simulink model "ValidateThrustersRED"  (R2020a)
settings: Solver=FixedStepAuto  StartTime=0.0  StopTime=tsim  RelTol=1e-3  EnableMultiTasking=on
undefined symbols (not defined in the file): Thruster1_OnTime, Thruster2_OnTime, Thruster3_OnTime, Thruster4_OnTime, Thruster5_OnTime, Thruster6_OnTime, Thruster7_OnTime, Thruster8_OnTime, ThrusterOff_Time
libraries: raspberrypiBasiclib x9
settings Model: SimulationMode=external  ExtModeTrigDuration=2  Creator=AlexC  LastModifiedBy=SPOT
settings SolverCC: PositivePriorityOrder=on
settings DataIOCC: ReturnWorkspaceOutputs=off
settings OptimizationCC: MaxStackSize=64
settings DebuggingCC: ParameterTunabilityLossMsg=error  ArithmeticOperatorsInVariantConditions=warning
settings HardwareCC: ProdBitPerPointer=32  ProdBitPerSizeT=32  ProdBitPerPtrDiffT=32  ProdLargestAtomicInteger=Long  ProdLargestAtomicFloat=Double  ProdWordSize=32  ProdHWDeviceType=ARM Compatible->ARM Cortex  UseEmbeddedCoderFeatures=off
settings SFSimCC: SimUseLocalCustomCode=off  CustomCodeUndefinedFunction=UseInterfaceOnly
settings RTWCC: SystemTargetFile=ert.tlc  HardwareBoard=Raspberry Pi  TemplateMakefile=ert_default_tmf  GenerateReport=on  RTWUseLocalCustomCode=off  Toolchain=GNU GCC Raspberry Pi  BuildConfiguration=Faster Runs  LaunchReport=on
settings CodeAppCC: ForceParamTrailComments=on  OperatorAnnotations=on  StateflowObjectComments=on  MATLABSourceComments=on
settings ERTTargetCC: ERTCustomFileBanners=off  MatFileLogging=on  SupportContinuousTime=on  SupportNonInlinedSFcns=on  RemoveResetFunc=off  SupportVariableSizeSignals=on  ModelStepFunctionPrototypeControlCompliant=off

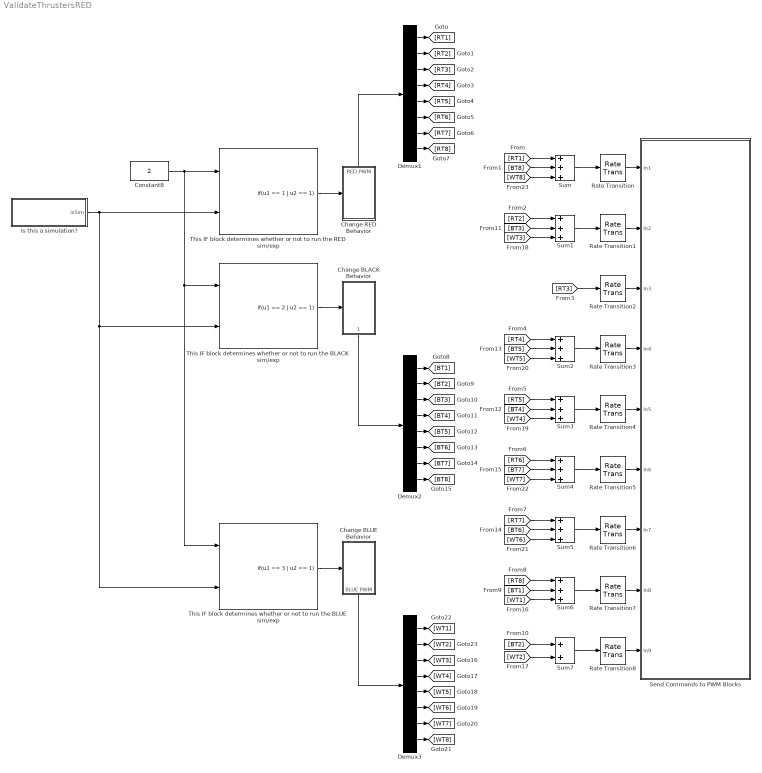
== system ValidateThrustersRED ==
  Change BLACK Behavior : Subsystem  TreatAsAtomicUnit=on
  Change BLUE Behavior : Subsystem  TreatAsAtomicUnit=on
  Change RED Behavior : Subsystem  TreatAsAtomicUnit=on
  Constant8 : Constant  Value=2
  Demux1 : Demux  Outputs=8
  Demux2 : Demux  Outputs=8
  Demux3 : Demux  Outputs=8
  Is this a simulation? : Subsystem
  Rate Transition{,1..8} (9 alike) : RateTransition  OutPortSampleTime=0.1
  Send Commands to PWM Blocks : Subsystem  TreatAsAtomicUnit=on  SystemSampleTime=0.1
  Sum{,1..6} (7 alike) : Sum  Inputs=+++
  Sum7 : Sum
  This IF block determines whether or not to run the BLACK sim/exp : If  NumInputs=2  IfExpression=u1 == 2 | u2 == 1  ShowElse=off
  This IF block determines whether or not to run the BLUE sim/exp : If  NumInputs=2  IfExpression=u1 == 3 | u2 == 1  ShowElse=off
  "This IF block determines whether or not to run the RED sim/exp " : If  NumInputs=2  IfExpression=u1 == 1 | u2 == 1  ShowElse=off
  wires:
  Demux3/8 -> [WT8]
  Rate Transition2/1 -> Send Commands to PWM Blocks/3(In3)
  Sum6/1 -> Rate Transition7/1
  This IF block determines whether or not to run the BLUE sim/exp/1 -> Change BLUE Behavior/Action
  Demux2/2 -> [BT2]
  This IF block determines whether or not to run the BLACK sim/exp/1 -> Change BLACK Behavior/Action
  Constant8/1 -> This IF block determines whether or not to run the BLUE sim/exp/1, This IF block determines whether or not to run the BLACK sim/exp/1, "This IF block determines whether or not to run the RED sim/exp "/1
  Demux2/4 -> [BT4]
  Rate Transition5/1 -> Send Commands to PWM Blocks/6(In6)
  Demux3/4 -> [WT4]
  Rate Transition8/1 -> Send Commands to PWM Blocks/9(In9)
  Demux3/7 -> [WT7]
  [RT4] -> Sum2/1
  Rate Transition7/1 -> Send Commands to PWM Blocks/8(In8)
  Sum4/1 -> Rate Transition5/1
  Demux1/7 -> [RT7]
  Demux3/6 -> [WT6]
  Demux1/8 -> [RT8]
  Demux1/3 -> [RT3]
  Sum3/1 -> Rate Transition4/1
  Sum5/1 -> Rate Transition6/1
  Sum2/1 -> Rate Transition3/1
  Change RED Behavior/1(RED PWM) -> Demux1/1
  [BT5] -> Sum2/2
  [BT7] -> Sum4/2
  [BT3] -> Sum1/2
  [RT2] -> Sum1/1
  [BT6] -> Sum5/2
  [BT8] -> Sum/2
  [RT7] -> Sum5/1
  Rate Transition3/1 -> Send Commands to PWM Blocks/4(In4)
  Change BLACK Behavior/1(BLACK PWM) -> Demux2/1
  Demux2/3 -> [BT3]
  Demux2/6 -> [BT6]
  Demux1/6 -> [RT6]
  [BT1] -> Sum6/2
  Demux2/7 -> [BT7]
  Demux1/4 -> [RT4]
  Is this a simulation?/1(isSim) -> This IF block determines whether or not to run the BLACK sim/exp/2, This IF block determines whether or not to run the BLUE sim/exp/2, "This IF block determines whether or not to run the RED sim/exp "/2
  Rate Transition4/1 -> Send Commands to PWM Blocks/5(In5)
  Demux2/5 -> [BT5]
  [WT3] -> Sum1/3
  Demux3/5 -> [WT5]
  Demux1/2 -> [RT2]
  [RT1] -> Sum/1
  [WT1] -> Sum6/3
  Demux3/3 -> [WT3]
  Sum/1 -> Rate Transition/1
  Sum7/1 -> Rate Transition8/1
  Demux2/8 -> [BT8]
  [RT8] -> Sum6/1
  [BT4] -> Sum3/2
  Change BLUE Behavior/1(BLUE PWM) -> Demux3/1
  Rate Transition6/1 -> Send Commands to PWM Blocks/7(In7)
  Demux1/5 -> [RT5]
  [RT5] -> Sum3/1
  Demux3/1 -> [WT1]
  Demux2/1 -> [BT1]
  [WT6] -> Sum5/3
  [WT2] -> Sum7/2
  "This IF block determines whether or not to run the RED sim/exp "/1 -> Change RED Behavior/Action
  [WT7] -> Sum4/3
  [RT6] -> Sum4/1
  [WT5] -> Sum2/3
  Sum1/1 -> Rate Transition1/1
  Demux3/2 -> [WT2]
  [BT2] -> Sum7/1
  [WT4] -> Sum3/3
  Demux1/1 -> [RT1]
  Rate Transition/1 -> Send Commands to PWM Blocks/1(In1)
  [WT8] -> Sum/3
  [RT3] -> Rate Transition2/1
  Rate Transition1/1 -> Send Commands to PWM Blocks/2(In2)

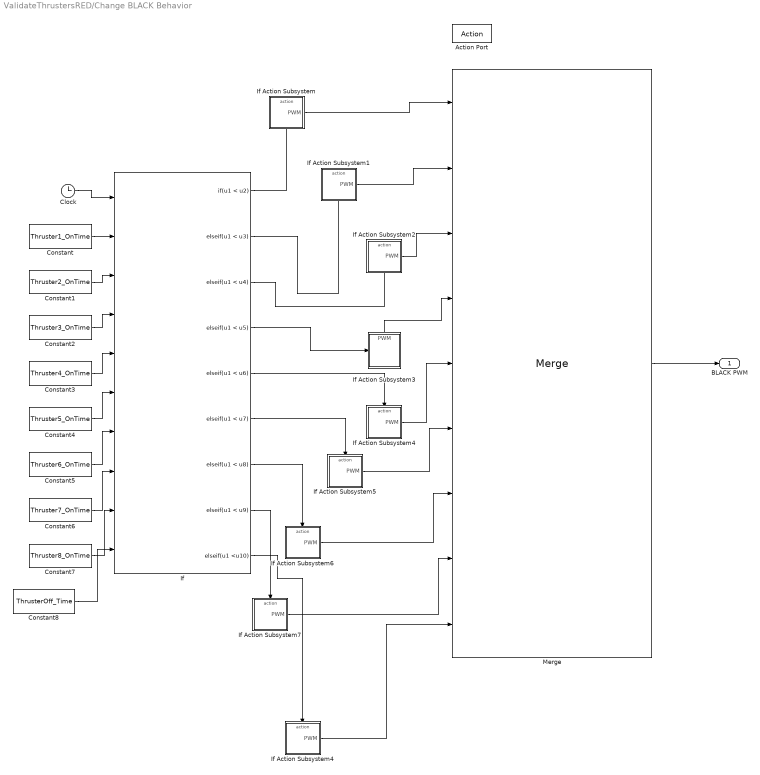
== system ValidateThrustersRED/Change BLACK Behavior ==
  Action Port : ActionPort  ActionPortLabel=if(u1 == 2 | u2 == 1)
  Clock : Clock
  Constant : Constant  Value=Thruster1_OnTime
  Constant1 : Constant  Value=Thruster2_OnTime
  Constant2 : Constant  Value=Thruster3_OnTime
  Constant3 : Constant  Value=Thruster4_OnTime
  Constant4 : Constant  Value=Thruster5_OnTime
  Constant5 : Constant  Value=Thruster6_OnTime
  Constant6 : Constant  Value=Thruster7_OnTime
  Constant7 : Constant  Value=Thruster8_OnTime
  Constant8 : Constant  Value=ThrusterOff_Time
  If : If  NumInputs=10  IfExpression=u1 < u2  ElseIfExpressions=u1 < u3, u1 < u4, u1 < u5, u1 < u6, u1 < u7, u1 < u8, u1 < u9, u1 <u10  ShowElse=off
  If Action Subsystem : Subsystem  TreatAsAtomicUnit=on
  If Action Subsystem1 : Subsystem  TreatAsAtomicUnit=on
  If Action Subsystem2 : Subsystem  TreatAsAtomicUnit=on
  If Action Subsystem3 : Subsystem  TreatAsAtomicUnit=on
  If Action Subsystem4 : Subsystem  TreatAsAtomicUnit=on
  If Action Subsystem5 : Subsystem  TreatAsAtomicUnit=on
  If Action Subsystem6 : Subsystem  TreatAsAtomicUnit=on
  If Action Subsystem7 : Subsystem  TreatAsAtomicUnit=on
  If Action Subsystem4 : Subsystem  TreatAsAtomicUnit=on
  Merge : Merge  Inputs=9
  BLACK PWM : Outport  VectorParamsAs1DForOutWhenUnconnected=off
  wires:
  Merge/1 -> BLACK PWM/1
  If/7 -> If Action Subsystem6/Action
  Constant6/1 -> If/8
  If/3 -> If Action Subsystem2/Action
  Constant4/1 -> If/6
  Constant3/1 -> If/5
  If Action Subsystem1/1(PWM) -> Merge/2
  If Action Subsystem2/1(PWM) -> Merge/3
  Constant/1 -> If/2
  Constant5/1 -> If/7
  Constant2/1 -> If/4
  If/5 -> If Action Subsystem4/Action
  If/6 -> If Action Subsystem5/Action
  If/8 -> If Action Subsystem7/Action
  Constant7/1 -> If/9
  If/2 -> If Action Subsystem1/Action
  If Action Subsystem4/1(PWM) -> Merge/5
  If Action Subsystem5/1(PWM) -> Merge/6
  If/4 -> If Action Subsystem3/Action
  If Action Subsystem/1(PWM) -> Merge/1
  If/1 -> If Action Subsystem/Action
  Clock/1 -> If/1
  Constant1/1 -> If/3
  If Action Subsystem6/1(PWM) -> Merge/7
  If Action Subsystem7/1(PWM) -> Merge/8
  If Action Subsystem3/1(PWM) -> Merge/4
  Constant8/1 -> If/10
  If Action Subsystem4/1(PWM) -> Merge/9
  If/9 -> If Action Subsystem4/Action

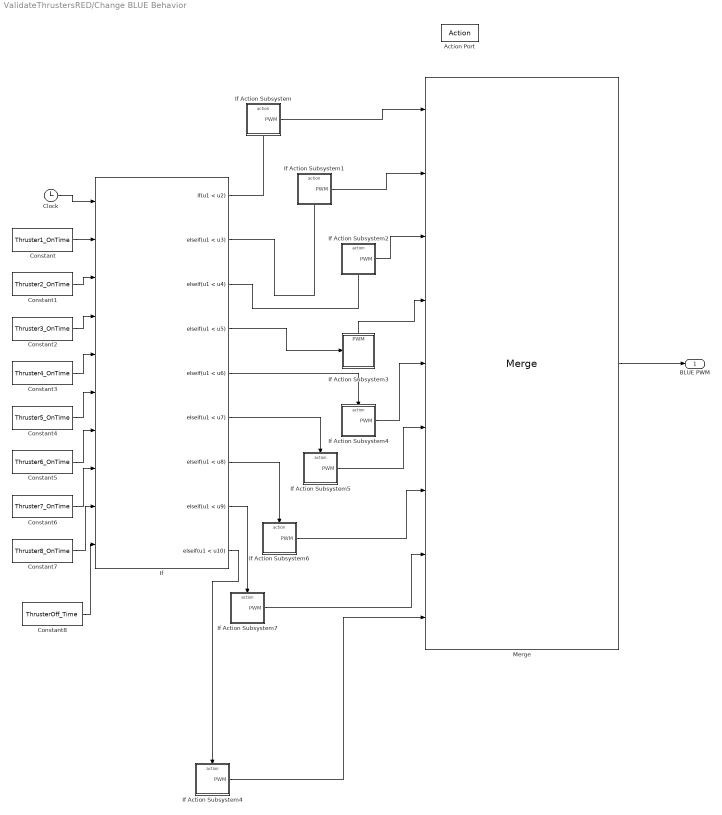
== system ValidateThrustersRED/Change BLUE Behavior ==
  Action Port : ActionPort  ActionPortLabel=if(u1 == 3 | u2 == 1)
  Clock : Clock
  Constant : Constant  Value=Thruster1_OnTime
  Constant1 : Constant  Value=Thruster2_OnTime
  Constant2 : Constant  Value=Thruster3_OnTime
  Constant3 : Constant  Value=Thruster4_OnTime
  Constant4 : Constant  Value=Thruster5_OnTime
  Constant5 : Constant  Value=Thruster6_OnTime
  Constant6 : Constant  Value=Thruster7_OnTime
  Constant7 : Constant  Value=Thruster8_OnTime
  Constant8 : Constant  Value=ThrusterOff_Time
  If : If  NumInputs=10  IfExpression=u1 < u2  ElseIfExpressions=u1 < u3, u1 < u4, u1 < u5, u1 < u6, u1 < u7, u1 < u8, u1 < u9, u1 < u10  ShowElse=off
  If Action Subsystem : Subsystem  TreatAsAtomicUnit=on
  If Action Subsystem1 : Subsystem  TreatAsAtomicUnit=on
  If Action Subsystem2 : Subsystem  TreatAsAtomicUnit=on
  If Action Subsystem3 : Subsystem  TreatAsAtomicUnit=on
  If Action Subsystem4 : Subsystem  TreatAsAtomicUnit=on
  If Action Subsystem5 : Subsystem  TreatAsAtomicUnit=on
  If Action Subsystem6 : Subsystem  TreatAsAtomicUnit=on
  If Action Subsystem7 : Subsystem  TreatAsAtomicUnit=on
  If Action Subsystem4 : Subsystem  TreatAsAtomicUnit=on
  Merge : Merge  Inputs=9
  BLUE PWM : Outport  VectorParamsAs1DForOutWhenUnconnected=off
  wires:
  Merge/1 -> BLUE PWM/1
  If/7 -> If Action Subsystem6/Action
  Constant6/1 -> If/8
  If/3 -> If Action Subsystem2/Action
  Constant4/1 -> If/6
  Constant3/1 -> If/5
  If Action Subsystem1/1(PWM) -> Merge/2
  If Action Subsystem2/1(PWM) -> Merge/3
  Constant/1 -> If/2
  Constant5/1 -> If/7
  Constant2/1 -> If/4
  If/5 -> If Action Subsystem4/Action
  If/6 -> If Action Subsystem5/Action
  If/8 -> If Action Subsystem7/Action
  Constant7/1 -> If/9
  If/2 -> If Action Subsystem1/Action
  If Action Subsystem4/1(PWM) -> Merge/5
  If Action Subsystem5/1(PWM) -> Merge/6
  If/4 -> If Action Subsystem3/Action
  If Action Subsystem/1(PWM) -> Merge/1
  If/1 -> If Action Subsystem/Action
  Clock/1 -> If/1
  Constant1/1 -> If/3
  If Action Subsystem6/1(PWM) -> Merge/7
  If Action Subsystem7/1(PWM) -> Merge/8
  If Action Subsystem3/1(PWM) -> Merge/4
  If Action Subsystem4/1(PWM) -> Merge/9
  If/9 -> If Action Subsystem4/Action
  Constant8/1 -> If/10

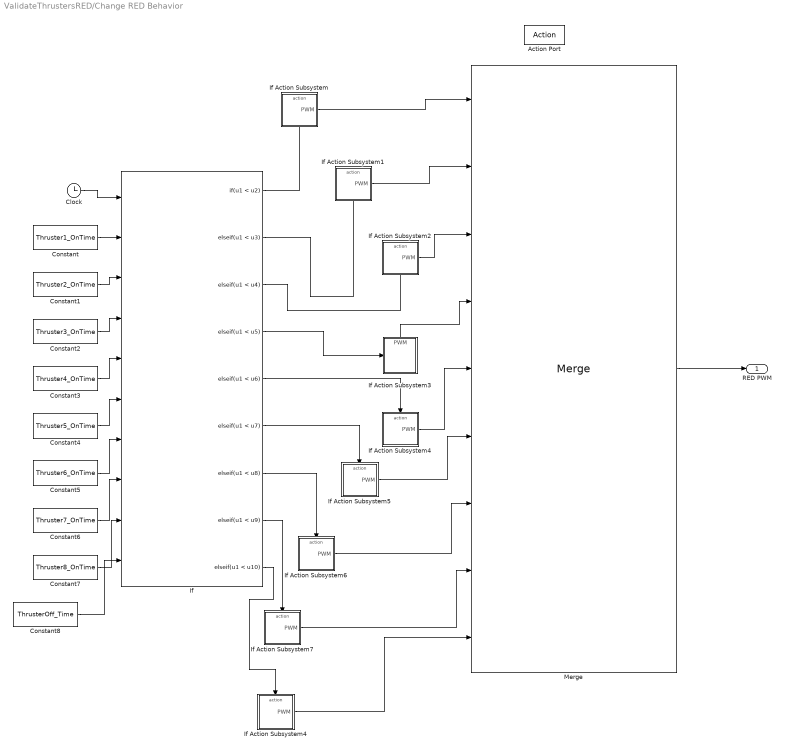
== system ValidateThrustersRED/Change RED Behavior ==
  Action Port : ActionPort  ActionPortLabel=if(u1 == 1 | u2 == 1)
  Clock : Clock
  Constant : Constant  Value=Thruster1_OnTime
  Constant1 : Constant  Value=Thruster2_OnTime
  Constant2 : Constant  Value=Thruster3_OnTime
  Constant3 : Constant  Value=Thruster4_OnTime
  Constant4 : Constant  Value=Thruster5_OnTime
  Constant5 : Constant  Value=Thruster6_OnTime
  Constant6 : Constant  Value=Thruster7_OnTime
  Constant7 : Constant  Value=Thruster8_OnTime
  Constant8 : Constant  Value=ThrusterOff_Time
  If : If  NumInputs=10  IfExpression=u1 < u2  ElseIfExpressions=u1 < u3, u1 < u4, u1 < u5, u1 < u6, u1 < u7, u1 < u8, u1 < u9, u1 < u10  ShowElse=off
  If Action Subsystem : Subsystem  TreatAsAtomicUnit=on
  If Action Subsystem1 : Subsystem  TreatAsAtomicUnit=on
  If Action Subsystem2 : Subsystem  TreatAsAtomicUnit=on
  If Action Subsystem3 : Subsystem  TreatAsAtomicUnit=on
  If Action Subsystem4 : Subsystem  TreatAsAtomicUnit=on
  If Action Subsystem5 : Subsystem  TreatAsAtomicUnit=on
  If Action Subsystem6 : Subsystem  TreatAsAtomicUnit=on
  If Action Subsystem7 : Subsystem  TreatAsAtomicUnit=on
  If Action Subsystem4 : Subsystem  TreatAsAtomicUnit=on
  Merge : Merge  Inputs=9
  RED PWM : Outport  VectorParamsAs1DForOutWhenUnconnected=off
  wires:
  Merge/1 -> RED PWM/1
  If/7 -> If Action Subsystem6/Action
  If Action Subsystem7/1(PWM) -> Merge/8
  If Action Subsystem3/1(PWM) -> Merge/4
  Constant1/1 -> If/3
  If Action Subsystem6/1(PWM) -> Merge/7
  Clock/1 -> If/1
  If/1 -> If Action Subsystem/Action
  If Action Subsystem4/1(PWM) -> Merge/5
  If Action Subsystem5/1(PWM) -> Merge/6
  If/4 -> If Action Subsystem3/Action
  If Action Subsystem/1(PWM) -> Merge/1
  Constant7/1 -> If/9
  If/6 -> If Action Subsystem5/Action
  If/5 -> If Action Subsystem4/Action
  If/8 -> If Action Subsystem7/Action
  Constant2/1 -> If/4
  Constant5/1 -> If/7
  Constant/1 -> If/2
  If Action Subsystem2/1(PWM) -> Merge/3
  If/2 -> If Action Subsystem1/Action
  If Action Subsystem1/1(PWM) -> Merge/2
  Constant3/1 -> If/5
  Constant4/1 -> If/6
  If/3 -> If Action Subsystem2/Action
  Constant6/1 -> If/8
  Constant8/1 -> If/10
  If/9 -> If Action Subsystem4/Action
  If Action Subsystem4/1(PWM) -> Merge/9

== system ValidateThrustersRED/Is this a simulation? ==
  Constant : Constant  Value=0  SampleTime=-1
  isSim : Outport  VectorParamsAs1DForOutWhenUnconnected=off
  wires:
  Constant/1 -> isSim/1

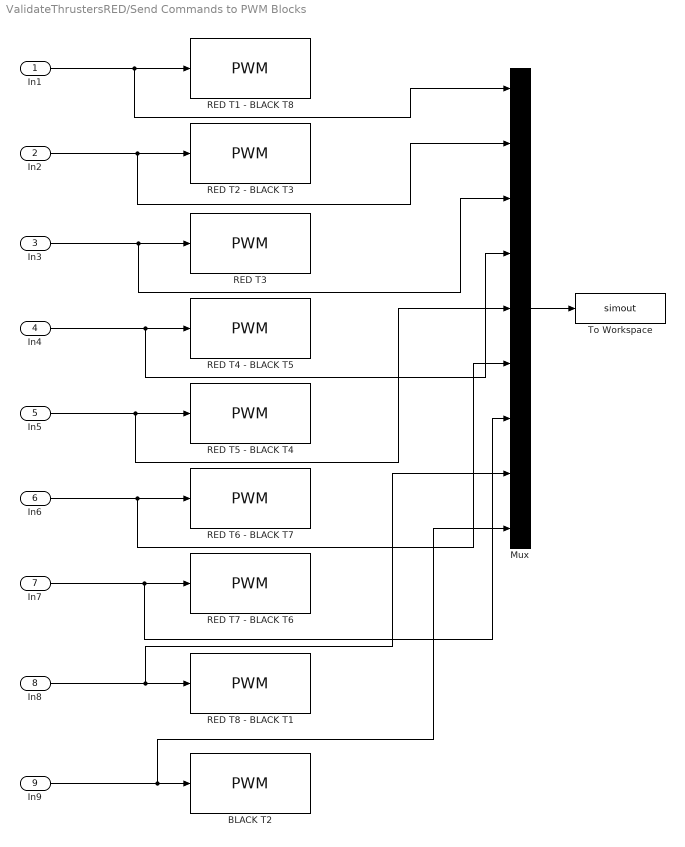
== system ValidateThrustersRED/Send Commands to PWM Blocks ==
  In1 : Inport
  In2 : Inport  Port=2
  In3 : Inport  Port=3
  In4 : Inport  Port=4
  In5 : Inport  Port=5
  In6 : Inport  Port=6
  In7 : Inport  Port=7
  In8 : Inport  Port=8
  In9 : Inport  Port=9
  BLACK T2 : raspberrypiBasiclib/PWM  board=Pi 3 Model B  Pin_=9  Frequency=10  blockPlatform=Raspberry Pi
      settings: SourceProductBaseCode=RASPPI
  Mux : Mux  Inputs=9
  RED T1 - BLACK T8 : raspberrypiBasiclib/PWM  board=Pi 3 Model B  Pin_=27  Frequency=10  blockPlatform=Raspberry Pi
      settings: SourceProductBaseCode=RASPPI
  RED T2 - BLACK T3 : raspberrypiBasiclib/PWM  board=Pi 3 Model B  Pin_=19  Frequency=10  blockPlatform=Raspberry Pi
      settings: SourceProductBaseCode=RASPPI
  RED T3 : raspberrypiBasiclib/PWM  board=Pi 3 Model B  Pin_=4  Frequency=10  blockPlatform=Raspberry Pi
      settings: SourceProductBaseCode=RASPPI
  RED T4 - BLACK T5 : raspberrypiBasiclib/PWM  board=Pi 3 Model B  Pin_=22  Frequency=10  blockPlatform=Raspberry Pi
      settings: SourceProductBaseCode=RASPPI
  RED T5 - BLACK T4 : raspberrypiBasiclib/PWM  board=Pi 3 Model B  Pin_=5  Frequency=10  blockPlatform=Raspberry Pi
      settings: SourceProductBaseCode=RASPPI
  RED T6 - BLACK T7 : raspberrypiBasiclib/PWM  board=Pi 3 Model B  Pin_=6  Frequency=10  blockPlatform=Raspberry Pi
      settings: SourceProductBaseCode=RASPPI
  RED T7 - BLACK T6 : raspberrypiBasiclib/PWM  board=Pi 3 Model B  Pin_=13  Frequency=10  blockPlatform=Raspberry Pi
      settings: SourceProductBaseCode=RASPPI
  RED T8 - BLACK T1 : raspberrypiBasiclib/PWM  board=Pi 3 Model B  Pin_=17  Frequency=10  blockPlatform=Raspberry Pi
      settings: SourceProductBaseCode=RASPPI
  To Workspace : ToWorkspace  VariableName=simout  SampleTime=-1
      settings: Save2DSignal=2-D array (concatenate along first dimension)
  wires:
  In4/1 -> Mux/4, RED T4 - BLACK T5/1
  In5/1 -> Mux/5, RED T5 - BLACK T4/1
  In1/1 -> Mux/1, RED T1 - BLACK T8/1
  In8/1 -> Mux/8, RED T8 - BLACK T1/1
  In9/1 -> Mux/9, BLACK T2/1
  In7/1 -> Mux/7, RED T7 - BLACK T6/1
  In6/1 -> Mux/6, RED T6 - BLACK T7/1
  In3/1 -> Mux/3, RED T3/1
  In2/1 -> Mux/2, RED T2 - BLACK T3/1
  Mux/1 -> To Workspace/1

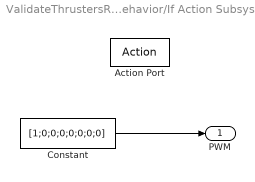
== system ValidateThrustersRED/Change BLACK Behavior/If Action Subsystem ==
  Action Port : ActionPort  ActionPortLabel=if(u1 < u2)
  Constant : Constant  Value=[1;0;0;0;0;0;0;0]
  PWM : Outport  VectorParamsAs1DForOutWhenUnconnected=off
  wires:
  Constant/1 -> PWM/1

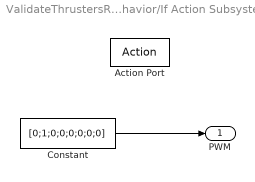
== system ValidateThrustersRED/Change BLACK Behavior/If Action Subsystem1 ==
  Action Port : ActionPort  ActionPortLabel=elseif(u1 < u3)
  Constant : Constant  Value=[0;1;0;0;0;0;0;0]
  PWM : Outport  VectorParamsAs1DForOutWhenUnconnected=off
  wires:
  Constant/1 -> PWM/1

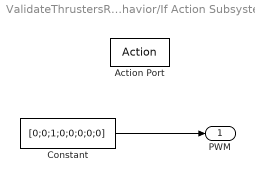
== system ValidateThrustersRED/Change BLACK Behavior/If Action Subsystem2 ==
  Action Port : ActionPort  ActionPortLabel=elseif( u1 < u4)
  Constant : Constant  Value=[0;0;1;0;0;0;0;0]
  PWM : Outport  VectorParamsAs1DForOutWhenUnconnected=off
  wires:
  Constant/1 -> PWM/1

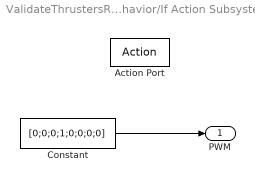
== system ValidateThrustersRED/Change BLACK Behavior/If Action Subsystem3 ==
  Action Port : ActionPort  ActionPortLabel=elseif( u1 < u5)
  Constant : Constant  Value=[0;0;0;1;0;0;0;0]
  PWM : Outport  VectorParamsAs1DForOutWhenUnconnected=off
  wires:
  Constant/1 -> PWM/1

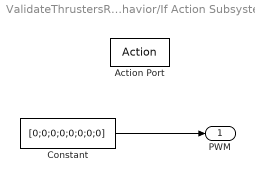
== system ValidateThrustersRED/Change BLACK Behavior/If Action Subsystem4 ==
  Action Port : ActionPort  ActionPortLabel=elseif( u1 <u10)
  Constant : Constant  Value=[0;0;0;0;0;0;0;0]
  PWM : Outport  VectorParamsAs1DForOutWhenUnconnected=off
  wires:
  Constant/1 -> PWM/1

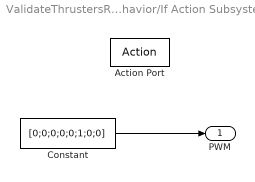
== system ValidateThrustersRED/Change BLACK Behavior/If Action Subsystem5 ==
  Action Port : ActionPort  ActionPortLabel=elseif( u1 < u7)
  Constant : Constant  Value=[0;0;0;0;0;1;0;0]
  PWM : Outport  VectorParamsAs1DForOutWhenUnconnected=off
  wires:
  Constant/1 -> PWM/1

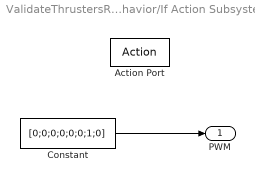
== system ValidateThrustersRED/Change BLACK Behavior/If Action Subsystem6 ==
  Action Port : ActionPort  ActionPortLabel=elseif( u1 < u8)
  Constant : Constant  Value=[0;0;0;0;0;0;1;0]
  PWM : Outport  VectorParamsAs1DForOutWhenUnconnected=off
  wires:
  Constant/1 -> PWM/1

== system ValidateThrustersRED/Change BLACK Behavior/If Action Subsystem7 ==
  Action Port : ActionPort  ActionPortLabel=elseif( u1 < u9)
  Constant : Constant  Value=[0;0;0;0;0;0;0;1]
  PWM : Outport  VectorParamsAs1DForOutWhenUnconnected=off
  wires:
  Constant/1 -> PWM/1

== system ValidateThrustersRED/Change BLACK Behavior/If Action Subsystem4 ==
  Action Port : ActionPort  ActionPortLabel=elseif( u1 < u6)
  Constant : Constant  Value=[0;0;0;0;1;0;0;0]
  PWM : Outport  VectorParamsAs1DForOutWhenUnconnected=off
  wires:
  Constant/1 -> PWM/1

== system ValidateThrustersRED/Change BLUE Behavior/If Action Subsystem ==
  Action Port : ActionPort  ActionPortLabel=if(u1 < u2)
  Constant : Constant  Value=[1;0;0;0;0;0;0;0]
  PWM : Outport  VectorParamsAs1DForOutWhenUnconnected=off
  wires:
  Constant/1 -> PWM/1

== system ValidateThrustersRED/Change BLUE Behavior/If Action Subsystem1 ==
  Action Port : ActionPort  ActionPortLabel=elseif(u1 < u3)
  Constant : Constant  Value=[0;1;0;0;0;0;0;0]
  PWM : Outport  VectorParamsAs1DForOutWhenUnconnected=off
  wires:
  Constant/1 -> PWM/1

== system ValidateThrustersRED/Change BLUE Behavior/If Action Subsystem2 ==
  Action Port : ActionPort  ActionPortLabel=elseif( u1 < u4)
  Constant : Constant  Value=[0;0;1;0;0;0;0;0]
  PWM : Outport  VectorParamsAs1DForOutWhenUnconnected=off
  wires:
  Constant/1 -> PWM/1

== system ValidateThrustersRED/Change BLUE Behavior/If Action Subsystem3 ==
  Action Port : ActionPort  ActionPortLabel=elseif( u1 < u5)
  Constant : Constant  Value=[0;0;0;1;0;0;0;0]
  PWM : Outport  VectorParamsAs1DForOutWhenUnconnected=off
  wires:
  Constant/1 -> PWM/1

== system ValidateThrustersRED/Change BLUE Behavior/If Action Subsystem4 ==
  Action Port : ActionPort  ActionPortLabel=elseif( u1 < u10)
  Constant : Constant  Value=[0;0;0;0;0;0;0;0]
  PWM : Outport  VectorParamsAs1DForOutWhenUnconnected=off
  wires:
  Constant/1 -> PWM/1

== system ValidateThrustersRED/Change BLUE Behavior/If Action Subsystem5 ==
  Action Port : ActionPort  ActionPortLabel=elseif( u1 < u7)
  Constant : Constant  Value=[0;0;0;0;0;1;0;0]
  PWM : Outport  VectorParamsAs1DForOutWhenUnconnected=off
  wires:
  Constant/1 -> PWM/1

== system ValidateThrustersRED/Change BLUE Behavior/If Action Subsystem6 ==
  Action Port : ActionPort  ActionPortLabel=elseif( u1 < u8)
  Constant : Constant  Value=[0;0;0;0;0;0;1;0]
  PWM : Outport  VectorParamsAs1DForOutWhenUnconnected=off
  wires:
  Constant/1 -> PWM/1

== system ValidateThrustersRED/Change BLUE Behavior/If Action Subsystem7 ==
  Action Port : ActionPort  ActionPortLabel=elseif( u1 < u9)
  Constant : Constant  Value=[0;0;0;0;0;0;0;1]
  PWM : Outport  VectorParamsAs1DForOutWhenUnconnected=off
  wires:
  Constant/1 -> PWM/1

== system ValidateThrustersRED/Change BLUE Behavior/If Action Subsystem4 ==
  Action Port : ActionPort  ActionPortLabel=elseif( u1 < u6)
  Constant : Constant  Value=[0;0;0;0;1;0;0;0]
  PWM : Outport  VectorParamsAs1DForOutWhenUnconnected=off
  wires:
  Constant/1 -> PWM/1

== system ValidateThrustersRED/Change RED Behavior/If Action Subsystem ==
  Action Port : ActionPort  ActionPortLabel=if(u1 < u2)
  Constant : Constant  Value=[1;0;0;0;0;0;0;0]
  PWM : Outport  VectorParamsAs1DForOutWhenUnconnected=off
  wires:
  Constant/1 -> PWM/1

== system ValidateThrustersRED/Change RED Behavior/If Action Subsystem1 ==
  Action Port : ActionPort  ActionPortLabel=elseif(u1 < u3)
  Constant : Constant  Value=[0;1;0;0;0;0;0;0]
  PWM : Outport  VectorParamsAs1DForOutWhenUnconnected=off
  wires:
  Constant/1 -> PWM/1

== system ValidateThrustersRED/Change RED Behavior/If Action Subsystem2 ==
  Action Port : ActionPort  ActionPortLabel=elseif( u1 < u4)
  Constant : Constant  Value=[0;0;1;0;0;0;0;0]
  PWM : Outport  VectorParamsAs1DForOutWhenUnconnected=off
  wires:
  Constant/1 -> PWM/1

== system ValidateThrustersRED/Change RED Behavior/If Action Subsystem3 ==
  Action Port : ActionPort  ActionPortLabel=elseif( u1 < u5)
  Constant : Constant  Value=[0;0;0;1;0;0;0;0]
  PWM : Outport  VectorParamsAs1DForOutWhenUnconnected=off
  wires:
  Constant/1 -> PWM/1

== system ValidateThrustersRED/Change RED Behavior/If Action Subsystem4 ==
  Action Port : ActionPort  ActionPortLabel=elseif( u1 < u10)
  Constant : Constant  Value=[0;0;0;0;0;0;0;0]
  PWM : Outport  VectorParamsAs1DForOutWhenUnconnected=off
  wires:
  Constant/1 -> PWM/1

== system ValidateThrustersRED/Change RED Behavior/If Action Subsystem5 ==
  Action Port : ActionPort  ActionPortLabel=elseif( u1 < u7)
  Constant : Constant  Value=[0;0;0;0;0;1;0;0]
  PWM : Outport  VectorParamsAs1DForOutWhenUnconnected=off
  wires:
  Constant/1 -> PWM/1

== system ValidateThrustersRED/Change RED Behavior/If Action Subsystem6 ==
  Action Port : ActionPort  ActionPortLabel=elseif( u1 < u8)
  Constant : Constant  Value=[0;0;0;0;0;0;1;0]
  PWM : Outport  VectorParamsAs1DForOutWhenUnconnected=off
  wires:
  Constant/1 -> PWM/1

== system ValidateThrustersRED/Change RED Behavior/If Action Subsystem7 ==
  Action Port : ActionPort  ActionPortLabel=elseif( u1 < u9)
  Constant : Constant  Value=[0;0;0;0;0;0;0;1]
  PWM : Outport  VectorParamsAs1DForOutWhenUnconnected=off
  wires:
  Constant/1 -> PWM/1

== system ValidateThrustersRED/Change RED Behavior/If Action Subsystem4 ==
  Action Port : ActionPort  ActionPortLabel=elseif( u1 < u6)
  Constant : Constant  Value=[0;0;0;0;1;0;0;0]
  PWM : Outport  VectorParamsAs1DForOutWhenUnconnected=off
  wires:
  Constant/1 -> PWM/1
